simulink model "BMS_Software_Harness1"  (R2022b)
settings: Solver=FixedStepDiscrete  StartTime=0.0  StopTime=5000  RelTol=1e-3
undefined symbols (not defined in the file): Ns_Module, NumModules
settings Model: DataDictionary=Shared_DD.sldd  EnableAccessToBaseWorkspace=off  PauseTimes=0  Creator=mluethy  LastModifiedBy=cpatel
settings SolverCC: AlgebraicLoopSolver=TrustRegion  PositivePriorityOrder=on  AutoInsertRateTranBlk=on
settings DataIOCC: ExternalInput=Battery  SaveOutput=off  SaveTime=off  SignalLoggingName=logsOut
settings OptimizationCC: BlockReduction=off  DefaultParameterBehavior=Inlined  UseFloatMulNetSlope=on  DefaultUnderspecifiedDataType=single  OptimizeBlockIOStorage=off  EnhancedBackFolding=on  PassReuseOutputArgsThreshold=0  ZeroExternalMemoryAtStartup=off  ZeroInternalMemoryAtStartup=off  EfficientFloat2IntCast=on  MaxStackSize=64  OptimizeBlockOrder=speed  DifferentSizesBufferReuse=on
settings DebuggingCC: SignalInfNanChecking=error  SaveWithParameterizedLinksMsg=none  CheckExecutionContextPreStartOutputMsg=on  IntegerOverflowMsg=error  ParameterPrecisionLossMsg=none  ParameterTunabilityLossMsg=error  UnconnectedInputMsg=warning  UnconnectedOutputMsg=warning  UnconnectedLineMsg=warning  AssertControl=DisableAll  PregeneratedLibrarySubsystemCodeDiagnostic=none  SFUnexpectedBacktrackingDiag=warning  SFNoUnconditionalDefaultTransitionDiag=warning  SFExecutionAtInitializationDiag=none  SFMachineParentedDataDiag=warning  ArithmeticOperatorsInVariantConditions=warning
settings HardwareCC: ProdBitPerLong=64  ProdLongLongMode=on  ProdHWDeviceType=Intel->x86-64 (Linux 64)
settings ModelReferenceCC: EnableRefExpFcnMdlSchedulingChecks=on  ModelReferenceNumInstancesAllowed=Single  PropagateSignalLabelsOutOfModel=off
settings SFSimCC: SimUseLocalCustomCode=off  MATLABDynamicMemAlloc=off  CustomCodeUndefinedFunction=UseInterfaceOnly
settings RTWCC: GenerateReport=on  RTWUseLocalCustomCode=off  Toolchain=Simulink Real-Time Toolchain  BuildConfiguration=Faster Runs  TargetLang=C++  DLArmComputeVersion=19.05
settings CodeAppCC: ForceParamTrailComments=on  MaxIdLength=51  OperatorAnnotations=on  MangleLength=4
settings GRTTargetCC: TargetLangStandard=C++03 (ISO)  CodeInterfacePackaging=C++ class
settings ConfigComp: CovMetricSettings=dcw  CovSaveCumulativeToWorkspaceVar=on  CovSaveSingleToWorkspaceVar=on  CovExternalEMLEnable=off  CovSFcnEnable=off  DVMode=DesignErrorDetection  DVMaxProcessTime=7000  DVTestSuiteOptimization=Auto  DVDetectDeadLogic=on  DVDetectIntegerOverflow=off  DVRebuildModelRepresentation=Always

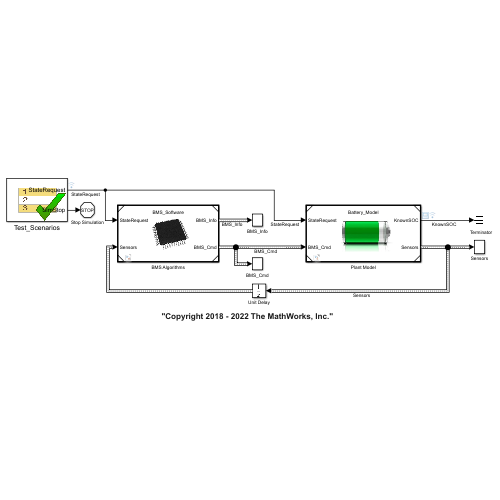
[thumbnail: Simulink's stored preview of the top-level diagram]
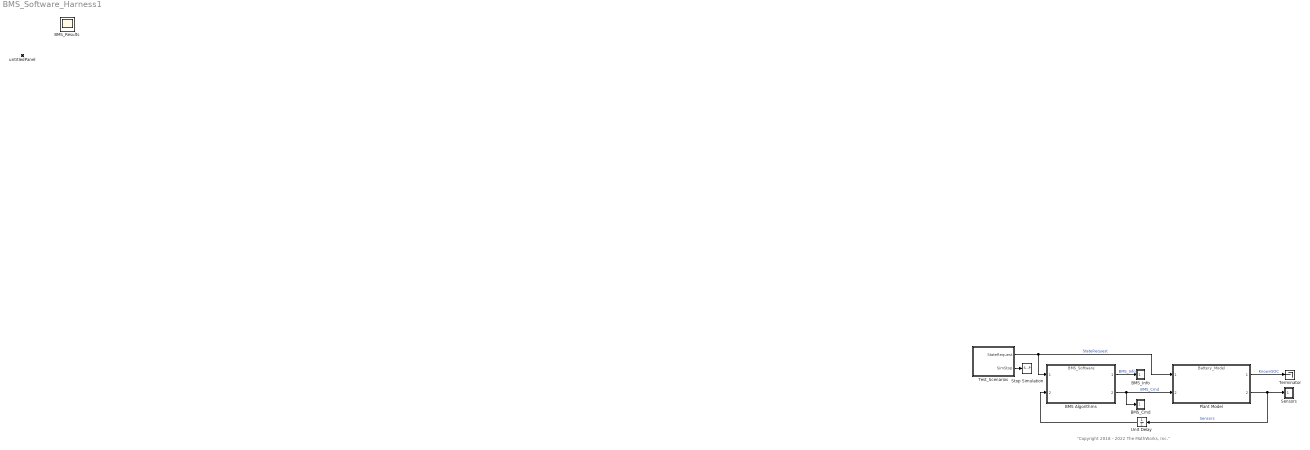
== system BMS_Software_Harness1 ==
  note: "Copyright 2018 - 2022 The MathWorks, Inc."
  BMS Algorithms : ModelReference  ModelNameDialog=BMS_Software  SimulationMode=Normal  ModelReferenceVersion=5.15
      mask Display: image('Microcontroller.jpg',[50,17,58,48])
  BMS_Cmd : Subsystem
  BMS_Info : Subsystem
  Plant Model : ModelReference  ModelNameDialog=Battery_Model  SimulationMode=Normal  ModelReferenceVersion=7.38
      mask Display: image('Plant_Battery.jpg',[50,15,80,48])
  Sensors : Subsystem
  Stop Simulation : Stop
  Terminator : Terminator
  Test_Scenarios : Test Sequence  TreatAsAtomicUnit=on  VariantControl=TestCase == 1
  Unit Delay : UnitDelay  InitialCondition=struct('Cell_Voltages',3.6*ones(1, Ns_Module*NumModules),'Pack_Voltage',3.6*Ns_Module*NumModules,'Pack_Current',0,'Cell_Temperatures',25*ones(1,Ns_Module*NumModules),'Vout_Chgr',0,'Vout_Invtr',0)  SampleTime=-1  HasFrameUpgradeWarning=on
  untitledPanel : Subsystem  Tag=HiddenForWebPanel  IsWebBlockPanel=on
  BMS_Results : Scope
  wires:
  BMS Algorithms/1 -> BMS_Info/1(BMS_Info)  "BMS_Info"
  BMS Algorithms/2 -> BMS_Cmd/1(In1), Plant Model/2  "BMS_Cmd"
  Plant Model/2 -> Sensors/1(" "), Unit Delay/1  "Sensors"
  Unit Delay/1 -> BMS Algorithms/2
  Test_Scenarios/1(StateRequest) -> Plant Model/1, BMS Algorithms/1  "StateRequest"
  Test_Scenarios/2(SimStop) -> Stop Simulation/1
  Plant Model/1 -> Terminator/1  "KnownSOC"

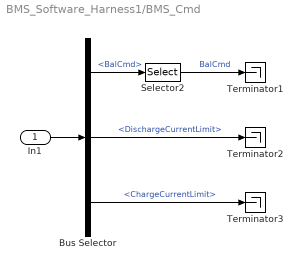
== system BMS_Software_Harness1/BMS_Cmd ==
  In1 : Inport
  Bus Selector : BusSelector  OutputSignals=BalCmd,CurrentLimits_Bus.DischargeCurrentLimit,CurrentLimits_Bus.ChargeCurrentLimit
  Selector2 : Selector  InputPortWidth=NumModules*Ns_Module  IndexOptions=Index vector (dialog)  Indices=[1:6]  OutputSizes=1
  Terminator1 : Terminator
  Terminator2 : Terminator
  Terminator3 : Terminator
  wires:
  In1/1 -> Bus Selector/1
  Bus Selector/1 -> Selector2/1  "<BalCmd>"
  Bus Selector/2 -> Terminator2/1  "<DischargeCurrentLimit>"
  Bus Selector/3 -> Terminator3/1  "<ChargeCurrentLimit>"
  Selector2/1 -> Terminator1/1  "BalCmd"

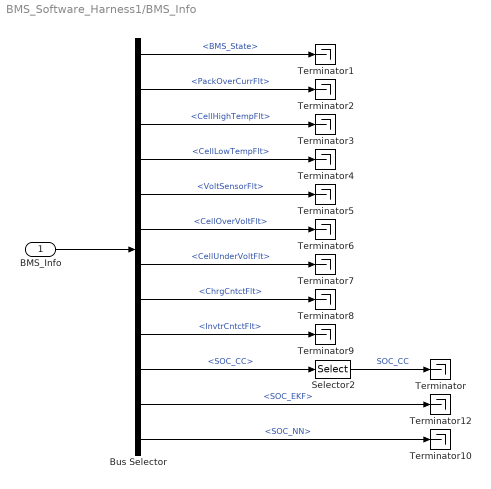
== system BMS_Software_Harness1/BMS_Info ==
  BMS_Info : Inport
  Bus Selector : BusSelector  OutputSignals=BMS_State,Faults_Bus.PackOverCurrFlt,Faults_Bus.CellHighTempFlt,Faults_Bus.CellLowTempFlt,Faults_Bus.VoltSensorFlt,Faults_Bus.CellOverVoltFlt,Faults_Bus.CellUnderVoltFlt,Faults_Bus.ChrgCntctFlt,Faults_Bus.InvtrCntctFlt,SOC.SOC_CC,SOC.SOC_EKF,SOC_NN
  Selector2 : Selector  InputPortWidth=NumModules*Ns_Module  IndexOptions=Index vector (dialog)  Indices=[1]  OutputSizes=1
  Terminator{,1..10,12} (12 alike) : Terminator
  wires:
  BMS_Info/1 -> Bus Selector/1
  Bus Selector/1 -> Terminator1/1  "<BMS_State>"
  Bus Selector/2 -> Terminator2/1  "<PackOverCurrFlt>"
  Bus Selector/3 -> Terminator3/1  "<CellHighTempFlt>"
  Bus Selector/4 -> Terminator4/1  "<CellLowTempFlt>"
  Bus Selector/5 -> Terminator5/1  "<VoltSensorFlt>"
  Bus Selector/6 -> Terminator6/1  "<CellOverVoltFlt>"
  Bus Selector/7 -> Terminator7/1  "<CellUnderVoltFlt>"
  Bus Selector/8 -> Terminator8/1  "<ChrgCntctFlt>"
  Bus Selector/9 -> Terminator9/1  "<InvtrCntctFlt>"
  Bus Selector/10 -> Selector2/1  "<SOC_CC>"
  Bus Selector/11 -> Terminator12/1  "<SOC_EKF>"
  Selector2/1 -> Terminator/1  "SOC_CC"
  Bus Selector/12 -> Terminator10/1  "<SOC_NN>"

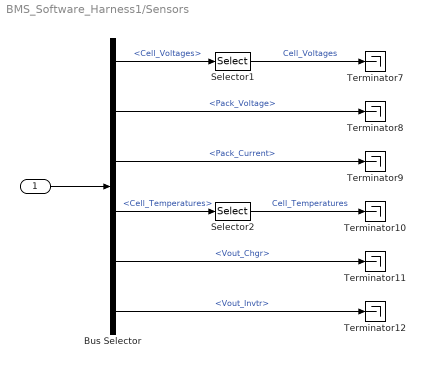
== system BMS_Software_Harness1/Sensors ==
  " " : Inport
  Bus Selector : BusSelector  OutputSignals=Cell_Voltages,Pack_Voltage,Pack_Current,Cell_Temperatures,Vout_Chgr,Vout_Invtr
  Selector1 : Selector  InputPortWidth=NumModules*Ns_Module  IndexOptions=Index vector (dialog)  Indices=[1:6]  OutputSizes=1
  Selector2 : Selector  InputPortWidth=NumModules*Ns_Module  IndexOptions=Index vector (dialog)  Indices=[1:6]  OutputSizes=1
  Terminator{7..12} (6 alike) : Terminator
  wires:
  Bus Selector/6 -> Terminator12/1  "<Vout_Invtr>"
  Bus Selector/5 -> Terminator11/1  "<Vout_Chgr>"
  Bus Selector/4 -> Selector2/1  "<Cell_Temperatures>"
  Bus Selector/3 -> Terminator9/1  "<Pack_Current>"
  Bus Selector/2 -> Terminator8/1  "<Pack_Voltage>"
  Bus Selector/1 -> Selector1/1  "<Cell_Voltages>"
  " "/1 -> Bus Selector/1
  Selector1/1 -> Terminator7/1  "Cell_Voltages"
  Selector2/1 -> Terminator10/1  "Cell_Temperatures"

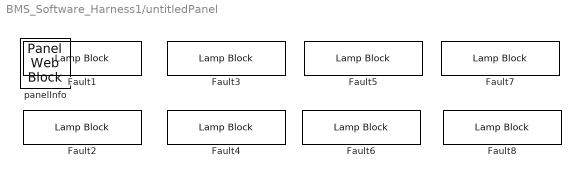
== system BMS_Software_Harness1/untitledPanel ==
  Fault1 : LampBlock  Tag=HiddenForWebPanel  PanelInfo="{\"height\":30,\"left\":15,\"panelId\":\"panelId-4b766684-a2de-49ad-8df5-635bc51aef69\",\"top\":16,\"type\":\"panelChild\",\"version\":\"2019b\",\"width\":102,\"zIndex\":1500014}"  Icon=Circle
  Fault2 : LampBlock  Tag=HiddenForWebPanel  PanelInfo="{\"height\":30,\"left\":15,\"panelId\":\"panelId-4b766684-a2de-49ad-8df5-635bc51aef69\",\"top\":76,\"type\":\"panelChild\",\"version\":\"2019b\",\"width\":102,\"zIndex\":1500012}"  Icon=Circle
  Fault3 : LampBlock  Tag=HiddenForWebPanel  PanelInfo="{\"height\":30,\"left\":140,\"panelId\":\"panelId-4b766684-a2de-49ad-8df5-635bc51aef69\",\"top\":16,\"type\":\"panelChild\",\"version\":\"2019b\",\"width\":102,\"zIndex\":1500002}"  Icon=Circle
  Fault4 : LampBlock  Tag=HiddenForWebPanel  PanelInfo="{\"height\":30,\"left\":140,\"panelId\":\"panelId-4b766684-a2de-49ad-8df5-635bc51aef69\",\"top\":76,\"type\":\"panelChild\",\"version\":\"2019b\",\"width\":102,\"zIndex\":1500004}"  Icon=Circle
  Fault5 : LampBlock  Tag=HiddenForWebPanel  PanelInfo="{\"height\":30,\"left\":259,\"panelId\":\"panelId-4b766684-a2de-49ad-8df5-635bc51aef69\",\"top\":16,\"type\":\"panelChild\",\"version\":\"2019b\",\"width\":102,\"zIndex\":1500008}"  Icon=Circle
  Fault6 : LampBlock  Tag=HiddenForWebPanel  PanelInfo="{\"height\":30,\"left\":258,\"panelId\":\"panelId-4b766684-a2de-49ad-8df5-635bc51aef69\",\"top\":76,\"type\":\"panelChild\",\"version\":\"2019b\",\"width\":102,\"zIndex\":1500006}"  Icon=Circle
  Fault7 : LampBlock  Tag=HiddenForWebPanel  PanelInfo="{\"height\":30,\"left\":378,\"panelId\":\"panelId-4b766684-a2de-49ad-8df5-635bc51aef69\",\"top\":16,\"type\":\"panelChild\",\"version\":\"2019b\",\"width\":102,\"zIndex\":1500010}"  Icon=Circle
  Fault8 : LampBlock  Tag=HiddenForWebPanel  PanelInfo="{\"height\":30,\"left\":380,\"panelId\":\"panelId-4b766684-a2de-49ad-8df5-635bc51aef69\",\"top\":76,\"type\":\"panelChild\",\"version\":\"2019b\",\"width\":102,\"zIndex\":1500016}"  Icon=Circle
  panelInfo : PanelWebBlock  Tag=HiddenForWebPanel  PanelInfo="{\"compacted\":false,\"height\":124,\"isActiveTab\":true,\"labels\":{},\"left\":320,\"name\":\"Panel\",\"panelId\":\"panelId-4b766684-a2de-49ad-8df5-635bc51aef69\",\"tabIndex\":0,\"tabbedSetId\":\"tabbedSet9399756491\",\"top\":16,\"type\":\"panel\",\"version\":\"2019b\",\"visible\":true,\"width\":501,\"zIndex\":1500002}"  PanelSnapshot=<binary blob, 12276 chars, not shown>

== stateflow chart BMS_Software_Harness1/Test_Scenarios ==
  state Driving_Charging_Rest
    state Driving
      StateRequest = SRE.Driving;
      SimStop = false;
    state Charging
      StateRequest = SRE.Charging;
    state Balancing
      StateRequest = SRE.Standby;
    state Stop
      SimStop = true;
    (default) -> Driving_Charging_Rest.Driving
    Driving_Charging_Rest.Driving -> Driving_Charging_Rest.Charging : [
        | after(2700,sec)
        | ]
    Driving_Charging_Rest.Charging -> Driving_Charging_Rest.Balancing : [
        | after(1800,sec)
        | ]
    Driving_Charging_Rest.Balancing -> Driving_Charging_Rest.Stop : [
        | after(500,sec)
        | ]
  state Charging
    state Charging
      StateRequest = SRE.Charging;
      SimStop = false;
    state Balancing
      StateRequest = SRE.Standby;
    state Stop
      SimStop = true;
    (default) -> Charging.Charging
    Charging.Charging -> Charging.Balancing : [
        | after(4200,sec)
        | ]
    Charging.Balancing -> Charging.Stop : [
        | after(1800,sec)
        | ]
  state Driving
    state Driving
      StateRequest = SRE.Driving;
      SimStop = false;
    state Balancing
      StateRequest = SRE.Standby;
    state Stop
      SimStop = true;
    (default) -> Driving.Driving
    Driving.Driving -> Driving.Balancing : [
        | after(8200,sec)
        | ]
    Driving.Balancing -> Driving.Stop : [
        | after(1500,sec)
        | ]
  (default) -> Driving_Charging_Rest [order 1] : [Active_Scenario_Index == 1]
  (default) -> Charging [order 2] : [Active_Scenario_Index == 2]
  (default) -> Driving [order 3] : {assert(Active_Scenario_Index == 3,'The value of Scenario Parameter ''Active_Scenario_Index'' is not valid. Use the index of the scenario to specify it.')}
  data: StateRequest output Enum: SRE; Active_Scenario_Index parameter; SimStop output
